simulink model "soc"  (R2026a)
settings: Solver=VariableStepAuto  StopTime=10.00

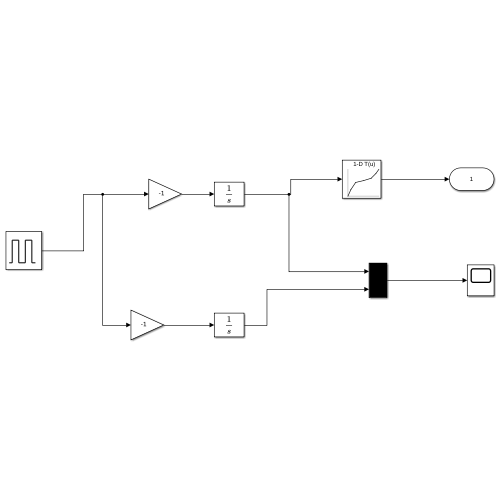
[thumbnail: Simulink's stored preview of the top-level diagram]
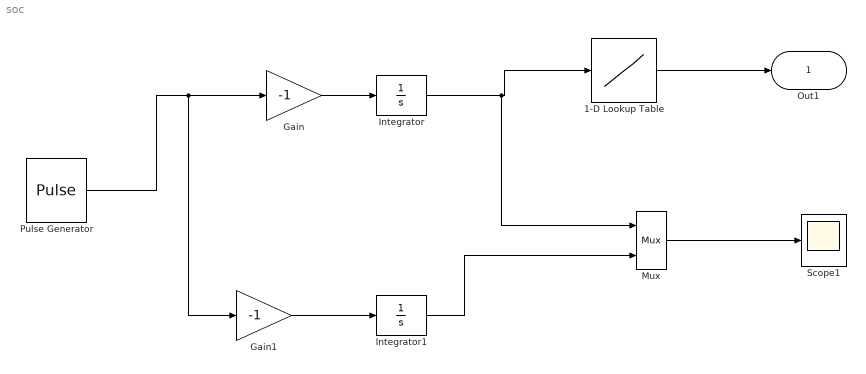
== system soc ==
  1-D Lookup Table : Lookup_n-D  NumberOfTableDimensions=1  BreakpointsForDimension1=[0, 0.1, 0.25, 0.5, 0.75, 0.9, 1.0]  Table=[3.0, 3.3, 3.6, 3.7, 3.8, 4.0, 4.2]  InternalRulePriority=Speed  RndMeth=Simplest
  Gain : Gain  Gain=-1
  Gain1 : Gain  Gain=-1
  Integrator : Integrator  InitialCondition=1
  Integrator1 : Integrator  InitialCondition=0.9
  Mux : Mux  Inputs=2
  Pulse Generator : DiscretePulseGenerator  PulseType=Time based  Amplitude=2  Period=10  PulseWidth=50
  Scope1 : Scope
      settings: ActiveDisplayYMinimum=-10.362499999999997  ActiveDisplayYMaximum=2.2624999999999993
  Out1 : Outport
  wires:
  Gain/1 -> Integrator/1
  Integrator/1 -> Mux/1, 1-D Lookup Table/1
  Integrator1/1 -> Mux/2
  1-D Lookup Table/1 -> Out1/1
  Pulse Generator/1 -> Gain1/1, Gain/1
  Mux/1 -> Scope1/1
  Gain1/1 -> Integrator1/1
